simulink model "bounce_simulink1"  (Simulink 4.1.1)
settings: Solver=ode23  SolverMode=SingleTasking  StartTime=0.0  StopTime=20  MaxStep=.01  RelTol=1e-3  AbsTol=1e-6
libraries: simulink3 x1
settings Model: Creator=monteiro  LastModifiedBy=jpk3  ExternalInput=[]  SaveTime=off  SaveOutput=off  InitialState=[]  LimitDataPoints=off  ExtModeTrigMode=oneshot  ExtModeArmWhenConnect=off

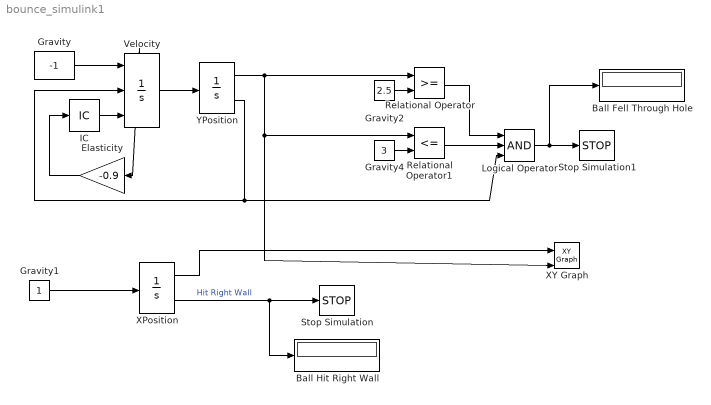
== system bounce_simulink1 ==
  Ball Fell Through Hole : Display
      settings: Format=short
  Ball Hit Right Wall : Display
      settings: Format=short
  Elasticity : Gain  Orientation=left  Gain=-0.9  Multiplication=Element-wise(K.*u)  SaturateOnIntegerOverflow=on
  Gravity : Constant  Value=-1
  Gravity1 : Constant  Value=1
  Gravity2 : Constant  Value=2.5
  Gravity4 : Constant  Value=3
  IC : InitialCondition  Value=0
  Logical Operator : Logic  Operator=AND  Inputs=3
  Relational Operator : RelationalOperator  Operator=>=
  Relational Operator1 : RelationalOperator  Operator=<=
  Stop Simulation : Stop
  Stop Simulation1 : Stop
  Velocity : Integrator  ExternalReset=falling  InitialConditionSource=external  InitialCondition=0  LimitOutput=off  UpperSaturationLimit=inf  LowerSaturationLimit=-inf  ShowSaturationPort=off  ShowStatePort=on  AbsoluteTolerance=auto
  XPosition : Integrator  ExternalReset=none  InitialConditionSource=internal  InitialCondition=0  LimitOutput=on  UpperSaturationLimit=4  LowerSaturationLimit=-inf  ShowSaturationPort=on  ShowStatePort=off  AbsoluteTolerance=auto
  XY Graph : simulink3/Sinks/XY Graph  xmin=0  xmax=5  ymin=0  ymax=3  st=-1
  YPosition : Integrator  ExternalReset=none  InitialConditionSource=internal  InitialCondition=1+sqrt(2)  LimitOutput=on  UpperSaturationLimit=inf  LowerSaturationLimit=1  ShowSaturationPort=on  ShowStatePort=off  AbsoluteTolerance=auto
  wires:
  Velocity/State -> Elasticity/1
  IC/1 -> Velocity/3
  Elasticity/1 -> IC/1
  Velocity/1 -> YPosition/1
  YPosition/1 -> Relational Operator1/1, XY Graph/2, Relational Operator/1
  Gravity/1 -> Velocity/1
  Gravity1/1 -> XPosition/1
  XPosition/2 -> Stop Simulation/1, Ball Hit Right Wall/1  "Hit Right Wall"
  Gravity2/1 -> Relational Operator/2
  Gravity4/1 -> Relational Operator1/2
  Relational Operator/1 -> Logical Operator/1
  Relational Operator1/1 -> Logical Operator/2
  Logical Operator/1 -> Stop Simulation1/1, Ball Fell Through Hole/1
  YPosition/2 -> Velocity/2, Logical Operator/3
  XPosition/1 -> XY Graph/1
